simulink model "ackerman_ROS_controller_obstaculos_2022"  (R2022b)
settings: Solver=FixedStepDiscrete  StartTime=0.0  StopTime=200  FixedStep=0.1  RelTol=1e-3
undefined symbols (not defined in the file or in its folder): Angular, Linear
libraries: robotlib x15, fuzblock x1, robotcorelib x1
settings Model: Creator=pizarro  LastModifiedBy=lublu
settings SolverCC: AlgebraicLoopSolver=TrustRegion
settings DebuggingCC: UnconnectedInputMsg=warning  UnconnectedOutputMsg=warning  UnconnectedLineMsg=warning
settings ModelReferenceCC: EnableRefExpFcnMdlSchedulingChecks=on
settings SFSimCC: CustomCodeUndefinedFunction=UseInterfaceOnly

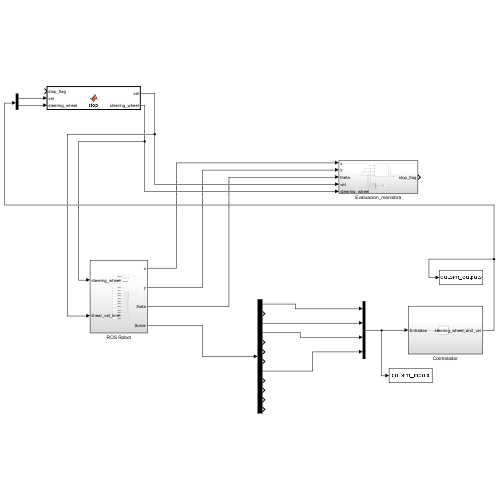
[thumbnail: Simulink's stored preview of the top-level diagram]
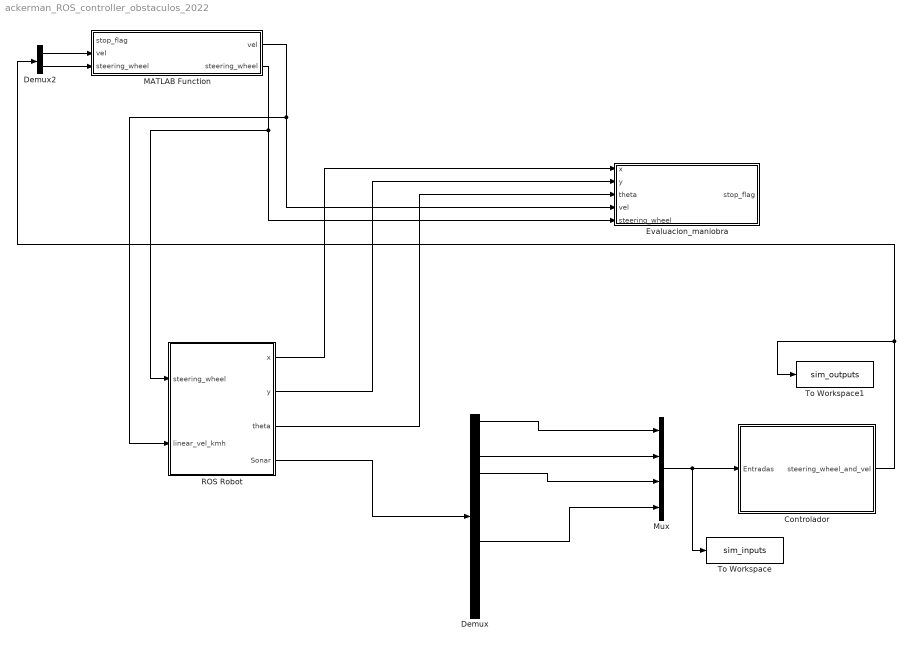
== system ackerman_ROS_controller_obstaculos_2022 ==
  Controlador : Subsystem
  Demux : Demux  Outputs=12
  Demux2 : Demux  Outputs=2
  Evaluacion_maniobra : Subsystem
  MATLAB Function : MATLAB Function  TreatAsAtomicUnit=on
  Mux : Mux
  ROS Robot : Subsystem
  To Workspace : ToWorkspace  VariableName=sim_inputs  SampleTime=-1
  To Workspace1 : ToWorkspace  VariableName=sim_outputs  SampleTime=-1
  wires:
  ROS Robot/1(x) -> Evaluacion_maniobra/1(x)
  ROS Robot/2(y) -> Evaluacion_maniobra/2(y)
  ROS Robot/3(theta) -> Evaluacion_maniobra/3(theta)
  Controlador/1(steering_wheel_and_vel) -> Demux2/1, To Workspace1/1
  MATLAB Function/1(vel) -> ROS Robot/2(linear_vel_kmh), Evaluacion_maniobra/4(vel)
  MATLAB Function/2(steering_wheel) -> Evaluacion_maniobra/5(steering_wheel), ROS Robot/1(steering_wheel)
  Demux2/1 -> MATLAB Function/2("vel ")
  Demux2/2 -> MATLAB Function/3("steering_wheel ")
  ROS Robot/4(Sonar) -> Demux/1
  Mux/1 -> To Workspace/1, Controlador/1(Entradas)
  Demux/1 -> Mux/1
  Demux/3 -> Mux/2
  Demux/4 -> Mux/3
  Demux/8 -> Mux/4

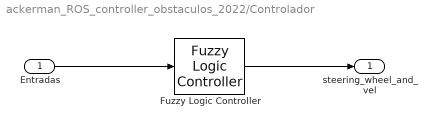
== system ackerman_ROS_controller_obstaculos_2022/Controlador ==
  Entradas : Inport
  Fuzzy Logic Controller : fuzblock/Fuzzy Logic  Controller  FIS='fuzzy_controller_obstaculos.fis'  OutputSampleNumber=101  DataType=double  FuzzifiedInputs=off  RuleFiringStrengths=off  RuleOutputs=off  AggregatedOutputs=off  SimulateUsing=Interpreted execution  OutOfRangeInputValueMessage=warning  NoRuleFiredMessage=warning  EmptyOutputFuzzySetMessage=warning
  steering_wheel_and_vel : Outport  VectorParamsAs1DForOutWhenUnconnected=off
  wires:
  Fuzzy Logic Controller/1 -> steering_wheel_and_vel/1
  Entradas/1 -> Fuzzy Logic Controller/1

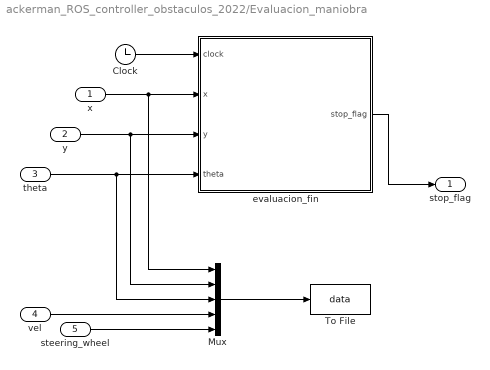
== system ackerman_ROS_controller_obstaculos_2022/Evaluacion_maniobra ==
  x : Inport
  y : Inport  Port=2
  theta : Inport  Port=3
  vel : Inport  Port=4
  steering_wheel : Inport  Port=5
  Clock : Clock
  Mux : Mux  Inputs=5
  To File : ToFile  Filename=data  MatrixName=data
  evaluacion_fin : MATLAB Function  TreatAsAtomicUnit=on
  stop_flag : Outport
  wires:
  theta/1 -> Mux/3, evaluacion_fin/4(theta)
  Clock/1 -> evaluacion_fin/1(clock)
  y/1 -> Mux/2, evaluacion_fin/3(y)
  evaluacion_fin/1(stop_flag) -> stop_flag/1
  Mux/1 -> To File/1
  x/1 -> Mux/1, evaluacion_fin/2(x)
  vel/1 -> Mux/4
  steering_wheel/1 -> Mux/5

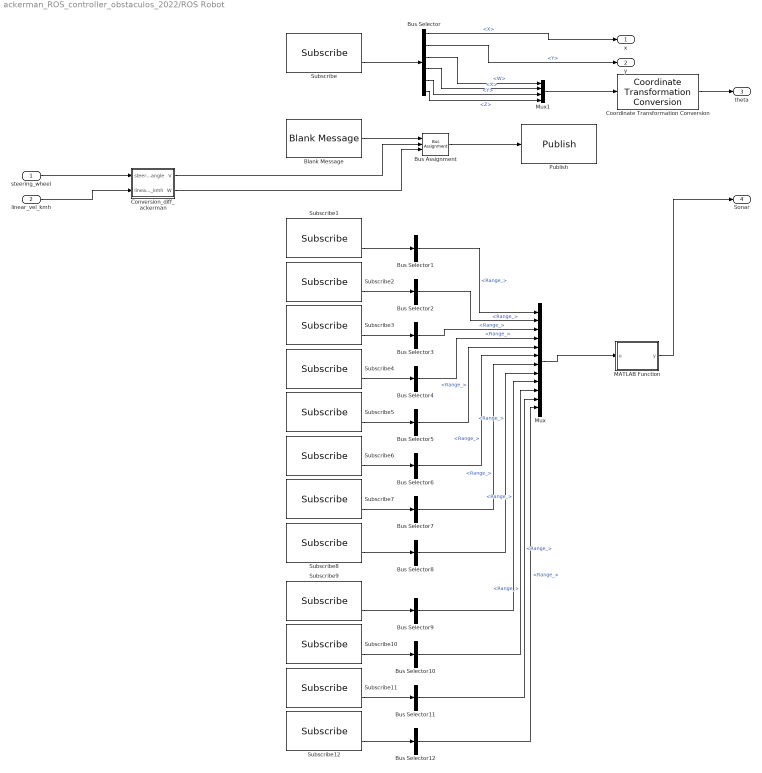
== system ackerman_ROS_controller_obstaculos_2022/ROS Robot ==
  steering_wheel : Inport
  linear_vel_kmh : Inport  Port=2
  Blank Message : robotlib/Blank Message  messageClass=Message  entityType=geometry_msgs/Twist  messageType=geometry_msgs/Twist  SampleTime=-1  legacyBusStruct=off
  Bus Assignment : BusAssignment  AssignedSignals=Linear.X,Angular.Z
  Bus Selector : BusSelector  OutputSignals=Pose.Pose.Position.X,Pose.Pose.Position.Y,Pose.Pose.Orientation.W,Pose.Pose.Orientation.X,Pose.Pose.Orientation.Y,Pose.Pose.Orientation.Z
  Bus Selector{1..12} (12 alike) : BusSelector  OutputSignals=Range_
  Conversion_diff_ackerman : MATLAB Function  TreatAsAtomicUnit=on
  Coordinate Transformation Conversion : robotcorelib/Coordinate Transformation Conversion  InputRepresentation=Quaternion  InputEulerSequence=ZYX  ShowTrVecInputPort=on  OutputRepresentation=Euler Angles  OutputEulerSequence=ZYX  ShowTrVecOutputPort=on  SimulateUsing=Interpreted execution
  MATLAB Function : MATLAB Function  TreatAsAtomicUnit=on
  Mux : Mux  Inputs=12
  Mux1 : Mux
  Publish : robotlib/Publish  topicSource=Select from ROS network  topic=/robot0/cmd_vel  messageType=geometry_msgs/Twist  legacyBusStruct=off  messageQueueLength=1
  Subscribe : robotlib/Subscribe  topicSource=Select from ROS network  topic=/robot0/odom  messageType=nav_msgs/Odometry  SampleTime=-1  legacyBusStruct=off  messageQueueLength=1
  Subscribe1 : robotlib/Subscribe  topicSource=Select from ROS network  topic=/robot0/sonar_0  messageType=sensor_msgs/Range  SampleTime=-1  legacyBusStruct=off  messageQueueLength=1
  Subscribe10 : robotlib/Subscribe  topicSource=Select from ROS network  topic=/robot0/sonar_9  messageType=sensor_msgs/Range  SampleTime=-1  legacyBusStruct=off  messageQueueLength=1
  Subscribe11 : robotlib/Subscribe  topicSource=Select from ROS network  topic=/robot0/sonar_10  messageType=sensor_msgs/Range  SampleTime=-1  legacyBusStruct=off  messageQueueLength=1
  Subscribe12 : robotlib/Subscribe  topicSource=Select from ROS network  topic=/robot0/sonar_11  messageType=sensor_msgs/Range  SampleTime=-1  legacyBusStruct=off  messageQueueLength=1
  Subscribe2 : robotlib/Subscribe  topicSource=Select from ROS network  topic=/robot0/sonar_1  messageType=sensor_msgs/Range  SampleTime=-1  legacyBusStruct=off  messageQueueLength=1
  Subscribe3 : robotlib/Subscribe  topicSource=Select from ROS network  topic=/robot0/sonar_2  messageType=sensor_msgs/Range  SampleTime=-1  legacyBusStruct=off  messageQueueLength=1
  Subscribe4 : robotlib/Subscribe  topicSource=Select from ROS network  topic=/robot0/sonar_3  messageType=sensor_msgs/Range  SampleTime=-1  legacyBusStruct=off  messageQueueLength=1
  Subscribe5 : robotlib/Subscribe  topicSource=Select from ROS network  topic=/robot0/sonar_4  messageType=sensor_msgs/Range  SampleTime=-1  legacyBusStruct=off  messageQueueLength=1
  Subscribe6 : robotlib/Subscribe  topicSource=Select from ROS network  topic=/robot0/sonar_5  messageType=sensor_msgs/Range  SampleTime=-1  legacyBusStruct=off  messageQueueLength=1
  Subscribe7 : robotlib/Subscribe  topicSource=Select from ROS network  topic=/robot0/sonar_6  messageType=sensor_msgs/Range  SampleTime=-1  legacyBusStruct=off  messageQueueLength=1
  Subscribe8 : robotlib/Subscribe  topicSource=Select from ROS network  topic=/robot0/sonar_7  messageType=sensor_msgs/Range  SampleTime=-1  legacyBusStruct=off  messageQueueLength=1
  Subscribe9 : robotlib/Subscribe  topicSource=Select from ROS network  topic=/robot0/sonar_8  messageType=sensor_msgs/Range  SampleTime=-1  legacyBusStruct=off  messageQueueLength=1
  x : Outport  VectorParamsAs1DForOutWhenUnconnected=off
  y : Outport  Port=2  VectorParamsAs1DForOutWhenUnconnected=off
  theta : Outport  Port=3  VectorParamsAs1DForOutWhenUnconnected=off
  Sonar : Outport  Port=4  VectorParamsAs1DForOutWhenUnconnected=off
  wires:
  Bus Selector/1 -> x/1  "<X>"
  Blank Message/1 -> Bus Assignment/1
  Subscribe/2 -> Bus Selector/1
  Bus Assignment/1 -> Publish/1
  Bus Selector/2 -> y/1  "<Y>"
  Subscribe1/2 -> Bus Selector1/1
  Conversion_diff_ackerman/1(V) -> Bus Assignment/2
  Conversion_diff_ackerman/2(W) -> Bus Assignment/3
  Subscribe2/2 -> Bus Selector2/1
  Subscribe3/2 -> Bus Selector3/1
  Subscribe5/2 -> Bus Selector5/1
  Subscribe4/2 -> Bus Selector4/1
  Subscribe6/2 -> Bus Selector6/1
  Subscribe7/2 -> Bus Selector7/1
  Bus Selector1/1 -> Mux/1  "<Range_>"
  Bus Selector2/1 -> Mux/2  "<Range_>"
  Bus Selector3/1 -> Mux/3  "<Range_>"
  Bus Selector4/1 -> Mux/4  "<Range_>"
  Bus Selector5/1 -> Mux/5  "<Range_>"
  Bus Selector6/1 -> Mux/6  "<Range_>"
  Bus Selector7/1 -> Mux/7  "<Range_>"
  Subscribe8/2 -> Bus Selector8/1
  Bus Selector8/1 -> Mux/8  "<Range_>"
  Bus Selector/3 -> Mux1/1  "<W>"
  Bus Selector/4 -> Mux1/2  "<X>"
  Bus Selector/5 -> Mux1/3  "<Y>"
  Bus Selector/6 -> Mux1/4  "<Z>"
  Mux1/1 -> Coordinate Transformation Conversion/1
  Coordinate Transformation Conversion/1 -> theta/1
  Mux/1 -> MATLAB Function/1(u)
  MATLAB Function/1(y) -> Sonar/1
  linear_vel_kmh/1 -> Conversion_diff_ackerman/2(linear_vel_ackerman_kmh)
  steering_wheel/1 -> Conversion_diff_ackerman/1(steering_wheel_angle)
  Subscribe9/2 -> Bus Selector9/1
  Bus Selector10/1 -> Mux/10  "<Range_>"
  Bus Selector9/1 -> Mux/9  "<Range_>"
  Bus Selector12/1 -> Mux/12  "<Range_>"
  Subscribe12/2 -> Bus Selector12/1
  Subscribe11/2 -> Bus Selector11/1
  Subscribe10/2 -> Bus Selector10/1
  Bus Selector11/1 -> Mux/11  "<Range_>"

== matlab function ackerman_ROS_controller_obstaculos_2022/ROS Robot/Conversion_diff_ackerman ==
  data: steering_wheel_angle input; V output; linear_vel_ackerman_kmh input; W output
function [V,W] = fcn(steering_wheel_angle, linear_vel_ackerman_kmh)

    %Aproximacion de angulo volante y velocidad linal a vel_linar y angular.
    % *************************************
    
    min_turning_radius_vehicle = 2;  % radio de giro del vehiculo. Radio minimo en el que gira 180 grados. 
    max_turning_radius_vehicle = 34; % radio de giro del vehiculo. Radio máximo con el volante girado 1º
    max_steering_wheel_angle = 90;  % angulo máximo de volante permitido (grados).
    max_vehicle_linear_speed = 50;  % velocidad máxima de vehiculo (km/h).
    
    
    % Filtrado des los valores máximos
    
    if steering_wheel_angle > max_steering_wheel_angle
        steering_wheel_angle = max_steering_wheel_angle;  
    end
    
    if steering_wheel_angle < (-1*max_steering_wheel_angle)
        steering_wheel_angle = max_steering_wheel_angle;  
    end
    
    if linear_vel_ackerman_kmh > max_vehicle_linear_speed
        linear_vel_ackerman_kmh = max_vehicle_linear_speed;
    end
    
    
    %Conversion a m/s
    linear_vel_ackerman_ms = linear_vel_ackerman_kmh/3.6; %(m/s)
    
    %Conversion a linear and angular velocity for the simulator.
    % v=rω --> ω = v/r
    
    % max_steering_wheel_angle -- > min_turning_radius_vehicle
    % steering_wheel_angle = 0 --> angular_vel_vehicle = 0;
    
    turning_radius = (max_turning_radius_vehicle-((max_turning_radius_vehicle-min_turning_radius_vehicle)/max_steering_wheel_angle)*abs(steering_wheel_angle));
    
    if steering_wheel_angle > 0
            turning_radius = turning_radius;
    elseif steering_wheel_angle < 0
            turning_radius = -1*turning_radius;
    end
    
    if abs(steering_wheel_angle) < 0.01
        angular_vel_vehicle = 0;
    else
        angular_vel_vehicle = linear_vel_ackerman_ms / turning_radius;
    end
    
    %Sin velocidad linear, tampoco debe girar
    
    if linear_vel_ackerman_ms == 0
        angular_vel_vehicle = 0;
    end
    
    
    %Rellenamos los campos del mensaje V y W
    V= linear_vel_ackerman_ms;

    W=angular_vel_vehicle;
    
    
    %********************************************************

== matlab function ackerman_ROS_controller_obstaculos_2022/ROS Robot/MATLAB Function ==
  data: u input; y output
function y = fcn(u)
u(isinf(u))=15.0;
y = u;

== matlab function ackerman_ROS_controller_obstaculos_2022/MATLAB Function ==
  data: stop_flag input; vel output; vel input; steering_wheel input; steering_wheel output
function [vel, steering_wheel]= stop(stop_flag,vel,steering_wheel)
    if stop_flag 
        steering_wheel=0;
        vel=0;
    else
        vel=vel;
        steering_wheel=steering_wheel;
    end

== matlab function ackerman_ROS_controller_obstaculos_2022/Evaluacion_maniobra/evaluacion_fin ==
  data: clock input; x input; y input; theta input; stop_flag output
function stop_flag = evaluacion_fin(clock, x, y, theta)
    if x > 59 && x < 60
        if y < 4
            stop_flag = 1;
        else 
            stop_flag = 0;
        end
        else
            stop_flag = 0;
    end
end
